simulink model "gyroboy_full"  (R2016b)
settings: Solver=FixedStepAuto  StartTime=0.0  StopTime=inf  FixedStep=Ts  RelTol=1e-3  EnableMultiTasking=on
PreLoadFcn:
  | config
  | preload
InitFcn:
  | plant
  | control
values from neighbouring files (symbols this model uses):
  A1 = [0 0   1 0 ... (first row only)    [plant.m]
  A2 = [0   1 ... (first row only)    [plant.m]
  B1 = [0 0 ... (first row only)    [plant.m]
  B2 = [0    0 ... (first row only)    [plant.m]
  C1 = eye(4)    [plant.m]
  C2 = eye(2)    [plant.m]
  D1 = zeros(4, 2)    [plant.m]
  D2 = zeros(2)    [plant.m]
  K = W / (2 * R) * alpha    [plant.m]
undefined symbols (not defined in the file or in its folder): DiscIntNeverNeededParam, K_PWM, Psi0, R, W
libraries: legoev3lib x5, simulink_extras x2, simulink x2
settings Model: SimulationMode=external  ExtModeTrigDuration=20000  Creator=roslovetspv  LastModifiedBy=roslovetspv
settings SolverCC: ZeroCrossAlgorithm=Adaptive  PositivePriorityOrder=on
settings OptimizationCC: MaxStackSize=64
settings DebuggingCC: ParameterTunabilityLossMsg=error
settings HardwareCC: ProdBitPerPointer=32  ProdBitPerSizeT=32  ProdBitPerPtrDiffT=32  ProdLargestAtomicInteger=Long  ProdWordSize=32  ProdHWDeviceType=ARM Compatible->ARM 9
settings RTWCC: SystemTargetFile=ert.tlc  HardwareBoard=LEGO MINDSTORMS EV3  TLCOptions="-aInlineSetEventsForThisBaseRateFcn=TLC_FALSE -aSuppressMultiTaskScheduler=TLC_FALSE  -aRateBasedStepFcn=0"  TemplateMakefile=ert_default_tmf  Description=Embedded Coder  GenerateReport=on  Toolchain=Sourcery G++ Lite v2009q3  IncludeHyperlinkInReport=on  LaunchReport=on  GenerateTraceInfo=on  GenerateTraceReport=on  GenerateTraceReportSl=on  GenerateTraceReportSf=on  GenerateTraceReportEml=on
settings CodeAppCC: ForceParamTrailComments=on  IgnoreCustomStorageClasses=off  OperatorAnnotations=on  SimulinkDataObjDesc=on  SFDataObjDesc=on  MATLABFcnDesc=on  InsertBlockDesc=on  MATLABSourceComments=on
settings ERTTargetCC: SupportContinuousTime=on  SupportVariableSizeSignals=on

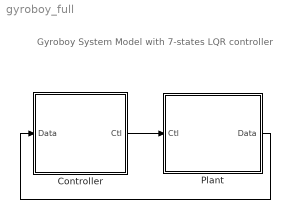
== system gyroboy_full ==
  note: Gyroboy System Model
      | with 7-states LQR controller
  Controller : Subsystem
  Plant : Subsystem  Variant=on  VariantControl=Variant1
  wires:
  Controller/1(Ctl) -> Plant/1("Ctl ")
  Plant/1(" Data") -> Controller/1(Data)

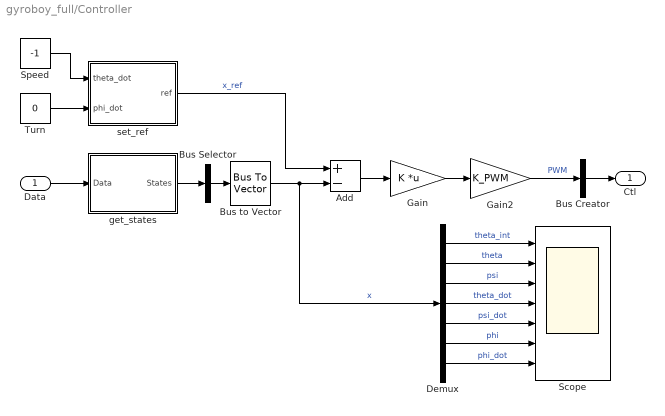
== system gyroboy_full/Controller ==
  Data : Inport
  Add : Sum  Inputs=+-
  Bus Creator : BusCreator  Inputs=1  OutDataTypeStr=Bus: Ctl
      settings: InheritFromInputs=off
  Bus Selector : BusSelector  OutputSignals=theta_int,theta,psi,theta_dot,psi_dot,phi,phi_dot  OutputAsBus=on
  Bus to Vector : BusToVector
  Demux : Demux  Outputs=7
  Gain : Gain  Gain=K  Multiplication=Matrix(K*u)
  Gain2 : Gain  Gain=K_PWM
  Scope : Scope  NumInputPorts=7
  Speed : Constant  Value=-1
  Turn : Constant  Value=0
  get_states : Subsystem
  set_ref : Subsystem
  Ctl : Outport
  wires:
  Bus Creator/1 -> Ctl/1
  Data/1 -> get_states/1(Data)
  get_states/1(States) -> Bus Selector/1
  Add/1 -> Gain/1
  Bus to Vector/1 -> Demux/1, Add/2  "x"
  Bus Selector/1 -> Bus to Vector/1
  Gain/1 -> Gain2/1
  Gain2/1 -> Bus Creator/1  "PWM"
  Speed/1 -> set_ref/1(theta_dot)
  Turn/1 -> set_ref/2(phi_dot)
  set_ref/1(ref) -> Add/1  "x_ref"
  Demux/1 -> Scope/1  "theta_int"
  Demux/2 -> Scope/2  "theta"
  Demux/3 -> Scope/3  "psi"
  Demux/4 -> Scope/4  "theta_dot"
  Demux/5 -> Scope/5  "psi_dot"
  Demux/6 -> Scope/6  "phi"
  Demux/7 -> Scope/7  "phi_dot"

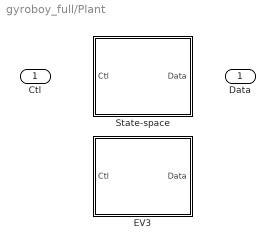
== system gyroboy_full/Plant ==
  "Ctl " : Inport
  EV3 : Subsystem  VariantControl=HW == 1
  State-space : Subsystem  VariantControl=(default)
  " Data" : Outport

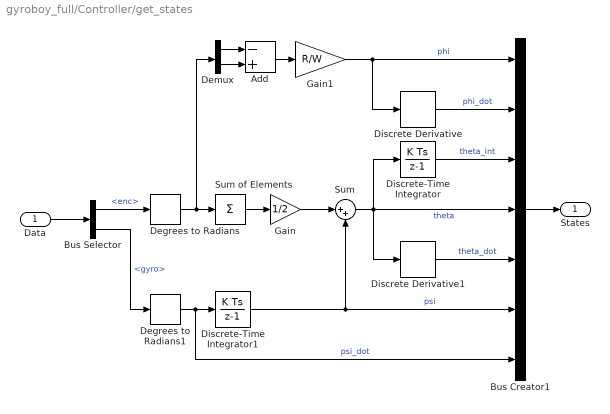
== system gyroboy_full/Controller/get_states ==
  Data : Inport
  Add : Sum  Inputs=-+
  Bus Creator1 : BusCreator  Inputs=7
  Bus Selector : BusSelector  OutputSignals=enc,gyro
  Degrees to Radians : simulink_extras/Transformations/Degrees to Radians
  Degrees to Radians1 : simulink_extras/Transformations/Degrees to Radians
  Demux : Demux  Outputs=2
  Discrete Derivative : simulink/Discrete/Discrete Derivative  gainval=1.0  ICPrevScaledInput=0.0  OutMin=[]  OutMax=[]  OutDataType=fixdt(1, 16)  OutScaling=2^-10  DoSatur=off
  Discrete Derivative1 : simulink/Discrete/Discrete Derivative  gainval=1.0  ICPrevScaledInput=0.0  OutMin=[]  OutMax=[]  OutDataType=fixdt(1, 16)  OutScaling=2^-10  DoSatur=off
  Discrete-Time Integrator : DiscreteIntegrator  InitialConditionSetting=State (most efficient)  SampleTime=-1  ICPrevOutput=DiscIntNeverNeededParam  ICPrevScaledInput=DiscIntNeverNeededParam
  Discrete-Time Integrator1 : DiscreteIntegrator  InitialConditionSetting=State (most efficient)  SampleTime=-1  ICPrevOutput=DiscIntNeverNeededParam  ICPrevScaledInput=DiscIntNeverNeededParam
  Gain : Gain  Gain=1/2
  Gain1 : Gain  Gain=R/W
  Sum : Sum  Inputs=|++
  Sum of Elements : Sum  Inputs=+
  States : Outport
  wires:
  Gain/1 -> Sum/1
  Degrees to Radians/1 -> Demux/1, Sum of Elements/1
  Discrete-Time Integrator1/1 -> Sum/2, Bus Creator1/6  "psi"
  Data/1 -> Bus Selector/1
  Bus Selector/1 -> Degrees to Radians/1  "<enc>"
  Sum/1 -> Discrete-Time Integrator/1, Discrete Derivative1/1, Bus Creator1/4  "theta"
  Discrete Derivative1/1 -> Bus Creator1/5  "theta_dot"
  Bus Creator1/1 -> States/1
  Sum of Elements/1 -> Gain/1
  Degrees to Radians1/1 -> Bus Creator1/7, Discrete-Time Integrator1/1  "psi_dot"
  Bus Selector/2 -> Degrees to Radians1/1  "<gyro>"
  Discrete-Time Integrator/1 -> Bus Creator1/3  "theta_int"
  Demux/1 -> Add/1
  Demux/2 -> Add/2
  Add/1 -> Gain1/1
  Gain1/1 -> Discrete Derivative/1, Bus Creator1/1  "phi"
  Discrete Derivative/1 -> Bus Creator1/2  "phi_dot"

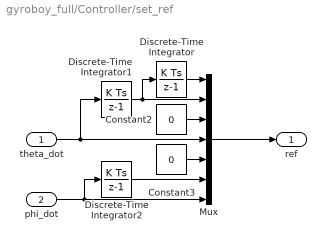
== system gyroboy_full/Controller/set_ref ==
  theta_dot : Inport
  phi_dot : Inport  Port=2
  Constant2 : Constant  Value=0
  Constant3 : Constant  Value=0
  Discrete-Time Integrator : DiscreteIntegrator  InitialConditionSetting=State (most efficient)  SampleTime=-1  ICPrevOutput=DiscIntNeverNeededParam  ICPrevScaledInput=DiscIntNeverNeededParam
  Discrete-Time Integrator1 : DiscreteIntegrator  InitialConditionSetting=State (most efficient)  SampleTime=-1  ICPrevOutput=DiscIntNeverNeededParam  ICPrevScaledInput=DiscIntNeverNeededParam
  Discrete-Time Integrator2 : DiscreteIntegrator  InitialConditionSetting=State (most efficient)  SampleTime=-1  ICPrevOutput=DiscIntNeverNeededParam  ICPrevScaledInput=DiscIntNeverNeededParam
  Mux : Mux  Inputs=7
  ref : Outport
  wires:
  Constant2/1 -> Mux/3
  Constant3/1 -> Mux/5
  Mux/1 -> ref/1
  Discrete-Time Integrator1/1 -> Discrete-Time Integrator/1, Mux/2
  phi_dot/1 -> Discrete-Time Integrator2/1, Mux/7
  Discrete-Time Integrator2/1 -> Mux/6
  Discrete-Time Integrator/1 -> Mux/1
  theta_dot/1 -> Discrete-Time Integrator1/1, Mux/4

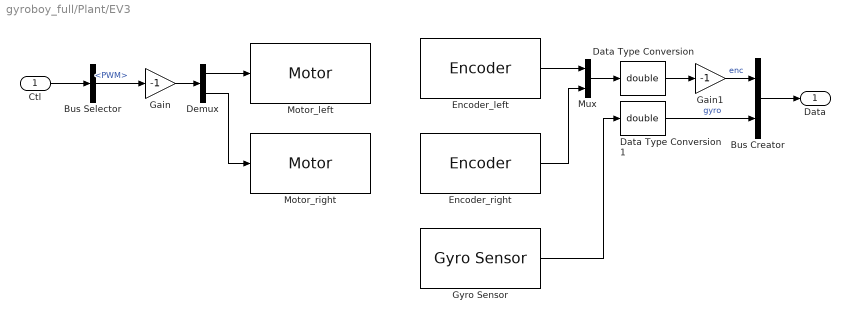
== system gyroboy_full/Plant/EV3 ==
  Ctl : Inport
  Bus Creator : BusCreator  Inputs=2
  Bus Selector : BusSelector  OutputSignals=PWM
  Data Type Conversion : DataTypeConversion  OutDataTypeStr=double
  Data Type Conversion1 : DataTypeConversion  OutDataTypeStr=double
  Demux : Demux  Outputs=2
  Encoder_left : legoev3lib/Encoder  portNumber=D  opMode=No reset  sampleTime=Ts
  Encoder_right : legoev3lib/Encoder  portNumber=A  opMode=No reset  sampleTime=Ts
  Gain : Gain  Gain=-1
  Gain1 : Gain  Gain=-1
  Gyro Sensor : legoev3lib/Gyro Sensor  portNumber=2  sampleTime=Ts
  Motor_left : legoev3lib/Motor  sportNumber=D  sstopAction=Brake
  Motor_right : legoev3lib/Motor  sportNumber=A  sstopAction=Brake
  Mux : Mux  Inputs=2
  Data : Outport
  wires:
  Ctl/1 -> Bus Selector/1
  Encoder_left/1 -> Mux/1
  Encoder_right/1 -> Mux/2
  Gyro Sensor/1 -> Data Type Conversion1/1
  Bus Selector/1 -> Gain/1  "<PWM>"
  Mux/1 -> Data Type Conversion/1
  Bus Creator/1 -> Data/1
  Demux/1 -> Motor_left/1
  Demux/2 -> Motor_right/1
  Gain/1 -> Demux/1
  Gain1/1 -> Bus Creator/1  "enc"
  Data Type Conversion/1 -> Gain1/1
  Data Type Conversion1/1 -> Bus Creator/2  "gyro"

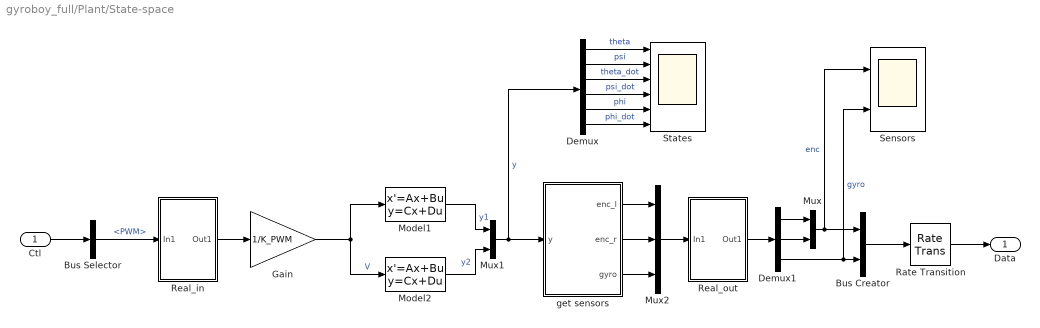
== system gyroboy_full/Plant/State-space ==
  Ctl : Inport
  Bus Creator : BusCreator  Inputs=2
  Bus Selector : BusSelector  OutputSignals=PWM
  Demux : Demux  Outputs=6
  Demux1 : Demux  Outputs=3
  Gain : Gain  Gain=1/K_PWM
  Model1 : StateSpace  A=A1  B=B1  C=C1  D=D1  X0=[0 Psi0 0 0]
  Model2 : StateSpace  A=A2  B=B2  C=C2  D=D2  X0=0
  Mux : Mux  Inputs=2
  Mux1 : Mux  Inputs=2
  Mux2 : Mux  Inputs=3
  Rate Transition : RateTransition  OutPortSampleTime=Ts
  Real_in : Subsystem  Variant=on  VariantControl=Variant1
  Real_out : Subsystem  Variant=on  VariantControl=Variant1
  Sensors : Scope  NumInputPorts=2
  States : Scope  NumInputPorts=6
  get sensors : MATLAB Function  TreatAsAtomicUnit=on
  Data : Outport
  wires:
  Model1/1 -> Mux1/1  "y1"
  Model2/1 -> Mux1/2  "y2"
  Gain/1 -> Model2/1, Model1/1  "V"
  Real_in/1(" Out1") -> Gain/1
  Ctl/1 -> Bus Selector/1
  Mux1/1 -> Demux/1, get sensors/1(y)  "y"
  Mux2/1 -> Real_out/1("In1 ")
  get sensors/3(gyro) -> Mux2/3
  Real_out/1(" Out1") -> Demux1/1
  Demux/4 -> States/4  "psi_dot"
  Demux/6 -> States/6  "phi_dot"
  Demux/5 -> States/5  "phi"
  Bus Creator/1 -> Rate Transition/1
  Demux1/1 -> Mux/1
  Demux1/2 -> Mux/2
  Demux1/3 -> Sensors/2, Bus Creator/2  "gyro"
  Demux/2 -> States/2  "psi"
  Demux/3 -> States/3  "theta_dot"
  Demux/1 -> States/1  "theta"
  Bus Selector/1 -> Real_in/1("In1 ")  "<PWM>"
  get sensors/1(enc_l) -> Mux2/1
  get sensors/2(enc_r) -> Mux2/2
  Mux/1 -> Sensors/1, Bus Creator/1  "enc"
  Rate Transition/1 -> Data/1

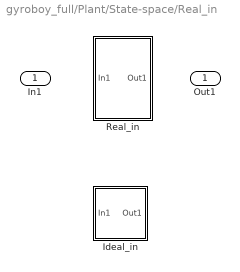
== system gyroboy_full/Plant/State-space/Real_in ==
  "In1 " : Inport
  Ideal_in : Subsystem  VariantControl=(default)
  Real_in : Subsystem  VariantControl=real_model == 1
  " Out1" : Outport

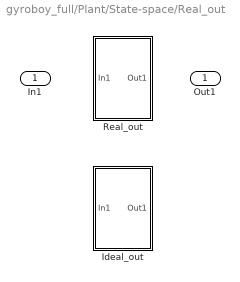
== system gyroboy_full/Plant/State-space/Real_out ==
  "In1 " : Inport
  Ideal_out : Subsystem  VariantControl=(default)
  Real_out : Subsystem  VariantControl=real_model == 1
  " Out1" : Outport

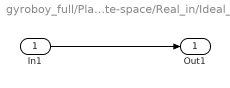
== system gyroboy_full/Plant/State-space/Real_in/Ideal_in ==
  "In1 " : Inport
  " Out1" : Outport
  wires:
  "In1 "/1 -> " Out1"/1

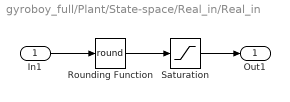
== system gyroboy_full/Plant/State-space/Real_in/Real_in ==
  In1 : Inport
  Rounding Function : Rounding  Operator=round
  Saturation : Saturate  UpperLimit=100  LowerLimit=-100
  Out1 : Outport
  wires:
  In1/1 -> Rounding Function/1
  Saturation/1 -> Out1/1
  Rounding Function/1 -> Saturation/1

== system gyroboy_full/Plant/State-space/Real_out/Ideal_out ==
  In1 : Inport
  Out1 : Outport
  wires:
  In1/1 -> Out1/1

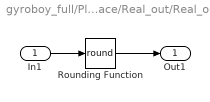
== system gyroboy_full/Plant/State-space/Real_out/Real_out ==
  In1 : Inport
  Rounding Function : Rounding  Operator=round
  Out1 : Outport
  wires:
  In1/1 -> Rounding Function/1
  Rounding Function/1 -> Out1/1

== matlab function gyroboy_full/Plant/State-space/get sensors ==
  data: enc_l output; enc_r output; y input; gyro output; R parameter; W parameter
function [enc_l, enc_r, gyro] = sensors(y, R, W)
enc_l = rad2deg(y(1) - W/R/2 * y(5) - y(2));
enc_r = rad2deg(y(1) + W/R/2 * y(5) - y(2));
gyro  = rad2deg(y(4));
